simulink model "video_test"  (R2018a)
settings: Solver=VariableStepAuto  StartTime=0.0  StopTime=inf  FixedStep=1/10  RelTol=1e-3
undefined symbols (not defined in the file): gray, none, videoinput
libraries: dspvision x1, imaqlib x1, simulink x1, PiCar_library x1
settings Model: Creator=Herib  LastModifiedBy=Herib

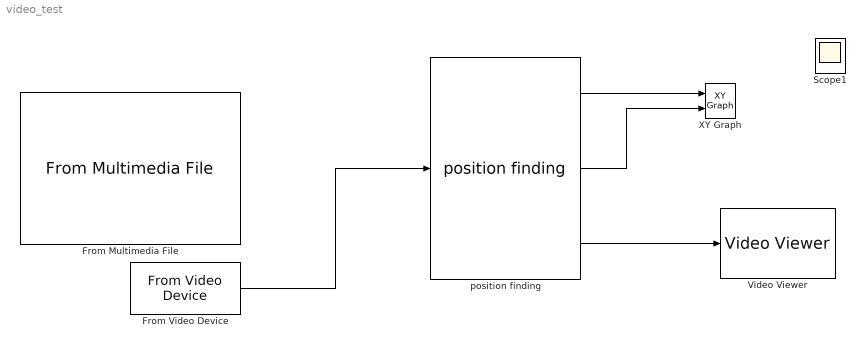
== system video_test ==
  From Multimedia File : dspvision/From Multimedia File  inputFilename=C:\Users\Herib\OneDrive\Bilder\Camera Roll\WIN_20181208_17_58_23_Pro.mp4  loop=on  numPlays=inf  outputStreams=Video only  videoDataType=single  audioDataType=int16  inheritSampleTime=on  userDefinedSampleTime=1/10  noAudioOutput=off  isIntensityVideo=off  fourcc=RGB  colorVideoFormat=One multidimensional signal  outputEOF=off  dataOrg=Column-major  audioFrameSize=1024  computeAudioFrameSize=off  outSamplingMode=Sample based
      settings: SourceProductBaseCode=VP
  From Video Device : imaqlib/From Video Device  DeviceMenu=winvideo 2 (Microsoft Camera Rear)  Device=winvideo 2 (Microsoft Camera Rear)  ObjConstructor=videoinput('winvideo', 2)  VideoFormatMenu=YUY2_640x480  VideoFormat=YUY2_640x480  VideoSource=input1  ROIPosition=[0 0 480 640]  EnableHWTrigger=off  TriggerConfiguration=none/none  SampleTime=1/30  OutputPortsMode=One multidimensional signal  DataType=single  CanDoHWTrigger=no  ReturnedColorSpace=rgb  BlockHandle=798.0033  ROIWidth=640  ROIHeight=480  ROIColumn=0  ROIRow=0  EngXMLPath=C:\Program Files\MATLAB\R2018a\toolbox\imaq\imaq\private  DevXMLPath=C:\ProgramData\MATLAB\SupportPackages\R2018a\toolbox\imaq\supportpackages\genericvideo\adaptor\win64  EngLibPath=C:\Program Files\MATLAB\R2018a\toolbox\imaq\imaqblks\imaqmex\win64  ColorSpace=rgb  BayerSensorAlignment=grbg
      settings: SourceProductName=Image Acquisition Toolbox
  Scope1 : Scope  NumInputPorts=2
  Video Viewer : VideoViewer  colormapValue=gray(256)  FigPos=[-744 527 714 591]
  XY Graph : simulink/Sinks/XY Graph  xmin=0  xmax=1  ymin=-0.5  ymax=0.5  st=1/10
  position finding : PiCar_library/position finding
      link override Selector: NumberOfDimensions=2
      link override Selector1: NumberOfDimensions=2
      link override Video Viewer: useColorMap=off  colormapValue=gray(256)  minInputVal=0  maxInputVal=255  specRange=off
      link override Video Viewer1: useColorMap=off  colormapValue=gray(256)  minInputVal=0  maxInputVal=255  specRange=off
      link override camera height: Value=0.21
  wires:
  position finding/3 -> Video Viewer/1
  position finding/1 -> XY Graph/1
  position finding/2 -> XY Graph/2
  From Video Device/1 -> position finding/1
